simulink model "interractorModelTutorial"  (R2018b)
settings: Solver=FixedStepAuto  StartTime=0.0  StopTime=3600*24  FixedStep=1  RelTol=1e-3
settings Model: Creator=cpp14rcj  LastModifiedBy=cpp14rcj

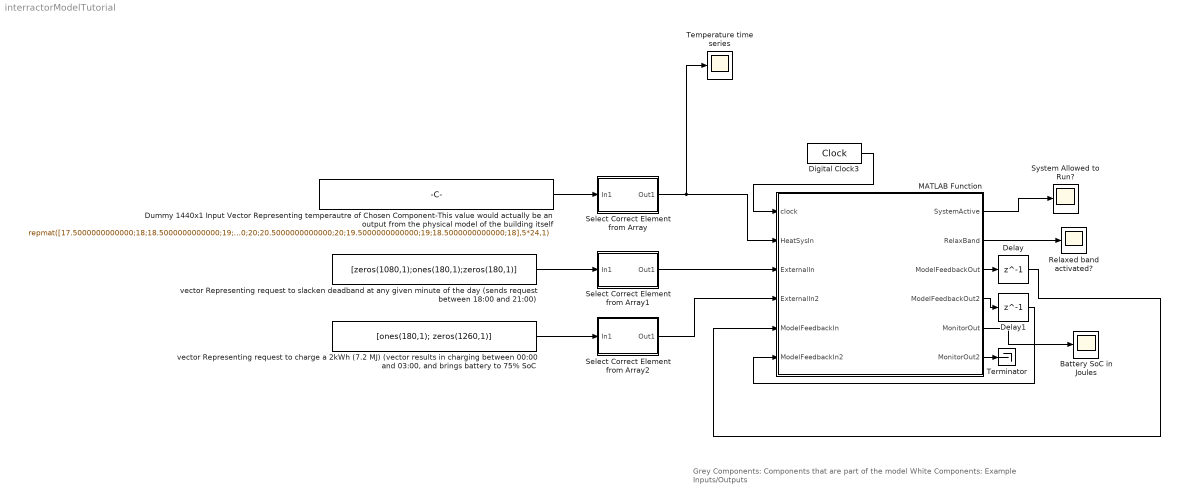
== system interractorModelTutorial ==
  note: Grey Components: Components that are part of the model
      | White Components: Example Inputs/Outputs
  Battery SoC in Joules : Scope
  Delay : Delay  DelayLength=1  InitialCondition=0
  Delay1 : Delay  DelayLength=1  InitialCondition=0
  Digital Clock3 : DigitalClock  SampleTime=5
  Dummy 1440x1 Input Vector Representing temperautre of Chosen Component-This value would actually be an output from the physical model of the building itself : Constant  Value=repmat([17.5000000000000;18;18.5000000000000;19;19.5000000000000;20;20.5000000000000;20;19.5000000000000;19;18.5000000000000;18],5*24,1)
  MATLAB Function : MATLAB Function  TreatAsAtomicUnit=on
  Relaxed band activated? : Scope
  Select Correct Element from Array : Subsystem
  Select Correct Element from Array1 : Subsystem
  Select Correct Element from Array2 : Subsystem
  System Allowed to Run? : Scope
  Temperature time series : Scope
  Terminator : Terminator
  "vector Representing request to charge a 2kWh (7.2 MJ) (vector results in charging between 00:00 and 03:00, and brings battery to 75% SoC" : Constant  Value=[ones(180,1); zeros(1260,1)]
  vector Representing request to slacken deadband at any given minute of the day (sends request between 18:00 and 21:00) : Constant  Value=[zeros(1080,1);ones(180,1);zeros(180,1)]
  wires:
  Delay/1 -> MATLAB Function/5(ModelFeedbackIn)
  MATLAB Function/1(SystemActive) -> System Allowed to Run?/1
  MATLAB Function/3(ModelFeedbackOut) -> Delay/1
  vector Representing request to slacken deadband at any given minute of the day (sends request between 18:00 and 21:00)/1 -> Select Correct Element from Array1/1(In1)
  MATLAB Function/2(RelaxBand) -> Relaxed band activated?/1
  "vector Representing request to charge a 2kWh (7.2 MJ) (vector results in charging between 00:00 and 03:00, and brings battery to 75% SoC"/1 -> Select Correct Element from Array2/1(In1)
  Select Correct Element from Array1/1(Out1) -> MATLAB Function/3(ExternalIn)
  Select Correct Element from Array2/1(Out1) -> MATLAB Function/4(ExternalIn2)
  MATLAB Function/4(ModelFeedbackOut2) -> Delay1/1
  Delay1/1 -> MATLAB Function/6(ModelFeedbackIn2)
  Digital Clock3/1 -> MATLAB Function/1(clock)
  Select Correct Element from Array/1(Out1) -> MATLAB Function/2(HeatSysIn), Temperature time series/1
  Dummy 1440x1 Input Vector Representing temperautre of Chosen Component-This value would actually be an output from the physical model of the building itself/1 -> Select Correct Element from Array/1(In1)
  MATLAB Function/6(MonitorOut2) -> Terminator/1
  MATLAB Function/5(MonitorOut) -> Battery SoC in Joules/1

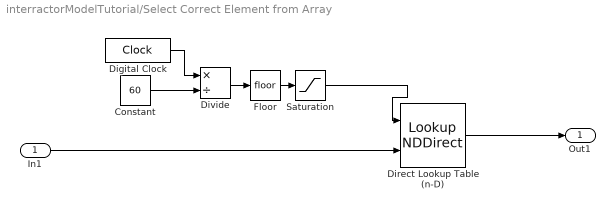
== system interractorModelTutorial/Select Correct Element from Array ==
  In1 : Inport
  Constant : Constant  Value=60
  Digital Clock : DigitalClock  SampleTime=5
  Direct Lookup Table (n-D) : LookupNDDirect  NumberOfTableDimensions=1  TableIsInput=on
  Divide : Product  Inputs=*/
  Floor : Rounding
  Saturation : Saturate  UpperLimit=1439  LowerLimit=0
  Out1 : Outport
  wires:
  Divide/1 -> Floor/1
  Saturation/1 -> Direct Lookup Table (n-D)/1
  Constant/1 -> Divide/2
  Floor/1 -> Saturation/1
  In1/1 -> Direct Lookup Table (n-D)/2
  Digital Clock/1 -> Divide/1
  Direct Lookup Table (n-D)/1 -> Out1/1

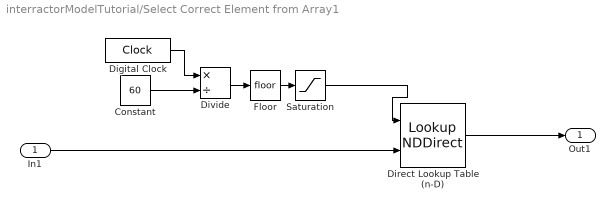
== system interractorModelTutorial/Select Correct Element from Array1 ==
  In1 : Inport
  Constant : Constant  Value=60
  Digital Clock : DigitalClock  SampleTime=5
  Direct Lookup Table (n-D) : LookupNDDirect  NumberOfTableDimensions=1  TableIsInput=on
  Divide : Product  Inputs=*/
  Floor : Rounding
  Saturation : Saturate  UpperLimit=1439  LowerLimit=0
  Out1 : Outport
  wires:
  Divide/1 -> Floor/1
  Saturation/1 -> Direct Lookup Table (n-D)/1
  Constant/1 -> Divide/2
  Floor/1 -> Saturation/1
  In1/1 -> Direct Lookup Table (n-D)/2
  Digital Clock/1 -> Divide/1
  Direct Lookup Table (n-D)/1 -> Out1/1

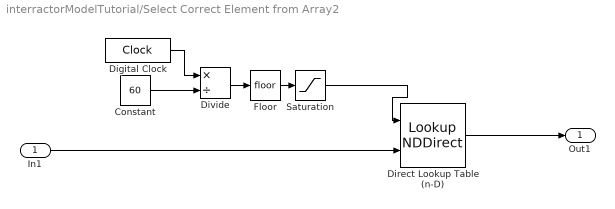
== system interractorModelTutorial/Select Correct Element from Array2 ==
  In1 : Inport
  Constant : Constant  Value=60
  Digital Clock : DigitalClock  SampleTime=5
  Direct Lookup Table (n-D) : LookupNDDirect  NumberOfTableDimensions=1  TableIsInput=on
  Divide : Product  Inputs=*/
  Floor : Rounding
  Saturation : Saturate  UpperLimit=1439  LowerLimit=0
  Out1 : Outport
  wires:
  Divide/1 -> Floor/1
  Saturation/1 -> Direct Lookup Table (n-D)/1
  Constant/1 -> Divide/2
  Floor/1 -> Saturation/1
  In1/1 -> Direct Lookup Table (n-D)/2
  Digital Clock/1 -> Divide/1
  Direct Lookup Table (n-D)/1 -> Out1/1

== matlab function interractorModelTutorial/MATLAB Function ==
  data: clock input; HeatSysIn input; SystemActive output; ExternalIn input; ExternalIn2 input; ModelFeedbackIn input; RelaxBand output; ModelFeedbackOut output; ModelFeedbackIn2 input; ModelFeedbackOut2 output; MonitorOut output; MonitorOut2 output
function [SystemActive,RelaxBand,ModelFeedbackOut,ModelFeedbackOut2,MonitorOut,MonitorOut2] = fcn(clock,HeatSysIn,ExternalIn,ExternalIn2,ModelFeedbackIn,ModelFeedbackIn2)

%INPUTS

%Clock - Inputs current simulation time
%
%HeatSys In - an input taken from the state of the building model e.g. the
%current temperature of one of the rooms, or the temperature of building
%component (e.g. wall or radiator). The user can manually change the input
%as shown in the instruction manual
%
%ExternalIn & ExternalIn2 - Time series inputs that are independent of
%model state, usually used to represent user of grid requests to turn
%systems on and off/ change thermostat settinggs
%
%ModelFeedbackIn & ModelFeedbackIn2 - Used to feed back a variable from the
%previous timestep, useful if updating variables such as State of Charge,
%or if latching a system on or off in a deadband (see example 1)

%OUTPUTS
%
%SystemActive -  variable that the user can control by programming logic in
%this function; deactivates heating system if set to zero, returns full control to
%default logic if set to 1. Routed to a scope in tutorial, Routed to space
%heating control in the real model.
%
%RelaxBand - binary variable that the user can control by programming logic in
%this function; changes the thermostat band to 16-16.1oC in the real model
%if set to 1,(minimum acceptable for thermal comfort) leaves thermostat band alone if set to zero.
%Routed to a scope in tutorial to show binary output.
%
%ModelFeedbackOut & ModelFeedbackOut2 - used to send variable values to the
%next timestep - useful when updating a variable such as state of charge,
%or latching a value when programming an additional thermostat (see example 1)

%% example 1  
%%Program for an additional space thermostat - 1440x1 matrix is used as
%%dummy input to represent temperature variation of the building component
%%(e.g. room/radiator) that we are controlling on

if HeatSysIn > 20  %e.g. if temp of chosen building compenent exceeds 20oC

SystemActive = 0; %switch off heating/keep heating off
ModelFeedbackOut=SystemActive; %send value to feedback out, so if temp is within deadband at next step, we can latch to the previous systemActive value

elseif HeatSysIn < 18 %if temp of chosen building compenent falls below 18oC

SystemActive = 1; %switch on heating/keep heating on
ModelFeedbackOut=SystemActive; %send value to feedback out, so if temp is within deadband at next step, we can latch to the previous systemActive value
    
else %if temp is within deadband
    
SystemActive = ModelFeedbackIn; %Latch to previous value i.e. if heating was on, keep it on, and vice versa
ModelFeedbackOut=SystemActive; %send value to feedback out, so if temp is within deadband at next step, we can latch to the previous systemActive value
    
end

%% example 2
%%use an externalIn array to read a value from a 1440x1 (1 element for each minute) binary vector
%%that reduces the thermostat temperature at times of high demand -
%%potentially useful for reduction in peak electricity demand

 
if ExternalIn == 1 %e.g. if external value is 1, which suggests band should be relaxed

RelaxBand=1; %Relax the space heating hysteresis band so that ower temps are acceptable

else

RelaxBand=0; %allow Heating System to continue running

end

%% example 3
%%charge a battery at 500W whenever a charge signal is recieved from the
%%1440x1 vector assigned to input 'ExternalIn1'

if clock == 0 %simulation is just starting
    
    StateOfCharge_J=0; %initialize SoC to zero
    ModelFeedbackOut2=StateOfCharge_J; %output for net timestep
    MonitorOut=StateOfCharge_J;
else

if ExternalIn2 == 1 && ModelFeedbackIn2 <7200000 %charge signal is being sent and store has not met 2kW limit
    
    StateOfCharge_J=ModelFeedbackIn2+500*5; %Charge Store at 500W (*5 accounts for 5 second timestep used by the model)
    ModelFeedbackOut2=StateOfCharge_J; %output new SoC
    MonitorOut=StateOfCharge_J;
else
    ModelFeedbackOut2=ModelFeedbackIn2; %State of Charge output is same as last timestep
    MonitorOut=ModelFeedbackOut2;
end
end

MonitorOut2=0; %set unused output to a fixed value
